simulink library "INT_Clth_VD"  (R2016b)
settings: Solver=VariableStepAuto  StartTime=0.0  StopTime=10.0  RelTol=1e-3
settings Model: Creator=Administrator  LastModifiedBy=Administrator

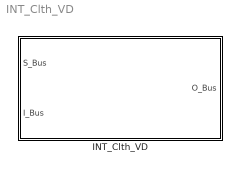
== system INT_Clth_VD ==
  INT_Clth_VD : Subsystem

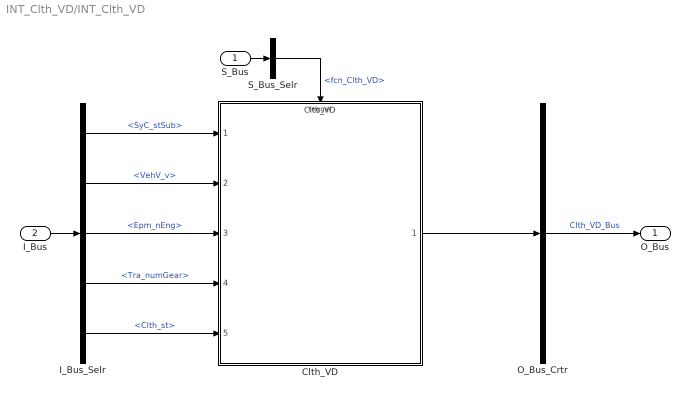
== system INT_Clth_VD/INT_Clth_VD ==
  S_Bus : Inport
  I_Bus : Inport  Port=2
  Clth_VD : ModelReference  ModelNameDialog=Clth_VD  SimulationMode=Normal  ModelReferenceVersion=1.9  TriggerPortName=function  TriggerPortTriggerType=function-call  TriggerPortStatesWhenEnabling=held
  I_Bus_Selr : BusSelector  OutputSignals=SyC_stSub,VehV_v,Epm_nEng,Tra_numGear,Clth_st
  O_Bus_Crtr : BusCreator  Inputs=1
  S_Bus_Selr : BusSelector  OutputSignals=fcn_Clth_VD
  O_Bus : Outport
  wires:
  S_Bus_Selr/1 -> Clth_VD/Trigger  "<fcn_Clth_VD>"
  S_Bus/1 -> S_Bus_Selr/1
  I_Bus/1 -> I_Bus_Selr/1
  I_Bus_Selr/1 -> Clth_VD/1  "<SyC_stSub>"
  I_Bus_Selr/2 -> Clth_VD/2  "<VehV_v>"
  I_Bus_Selr/3 -> Clth_VD/3  "<Epm_nEng>"
  I_Bus_Selr/4 -> Clth_VD/4  "<Tra_numGear>"
  I_Bus_Selr/5 -> Clth_VD/5  "<Clth_st>"
  O_Bus_Crtr/1 -> O_Bus/1  "Clth_VD_Bus"
  Clth_VD/1 -> O_Bus_Crtr/1
